simulink model "SafetyTemperatureSwitch"  (R2016b)
settings: Solver=FixedStepDiscrete  StartTime=0.0  StopTime=inf  RelTol=1e-3  EnableMultiTasking=on
settings Model: xpc_rtwmakecfg_data=_xpcethercatlib_  Creator=march  LastModifiedBy=march
settings SolverCC: EnableConcurrentExecution=on  AutoInsertRateTranBlk=on
settings DataIOCC: SaveFormat=StructureWithTime  SaveOutput=off  SaveTime=off
settings OptimizationCC: BlockReduction=off  OptimizeBlockIOStorage=off  BufferReuse=off  GlobalBufferReuse=off  ExpressionFolding=off  LocalBlockOutputs=off
settings HardwareCC: ProdBitPerPointer=32  ProdBitPerSizeT=32  ProdBitPerPtrDiffT=32  ProdLargestAtomicFloat=None  ProdWordSize=32  ProdLongLongMode=on  ProdHWDeviceType=Generic->32-bit x86 compatible
settings RTWCC: SystemTargetFile=slrt.tlc  TemplateMakefile=slrt_default_tmf  PostCodeGenCommand=SomanetTuning_make_rtw_hook  Description=Simulink Real-Time  RTWVerbose=off  CodeExecutionProfiling=on  RTWCompilerOptimization=on
settings SimulinkRealTimeCC: xPCModelTimeoutSecs=20

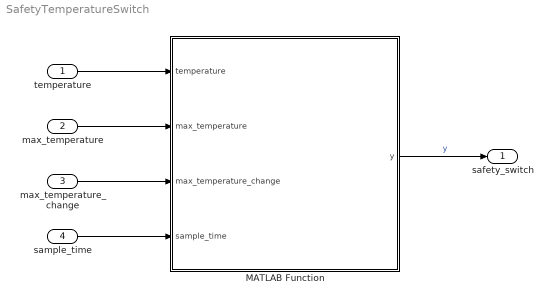
== system SafetyTemperatureSwitch ==
  "temperature " : Inport
  max_temperature : Inport  Port=2
  max_temperature_change : Inport  Port=3
  sample_time : Inport  Port=4
  MATLAB Function : MATLAB Function  TreatAsAtomicUnit=on
  safety_switch : Outport
  wires:
  sample_time/1 -> MATLAB Function/4(sample_time)
  max_temperature_change/1 -> MATLAB Function/3(max_temperature_change)
  max_temperature/1 -> MATLAB Function/2(max_temperature)
  "temperature "/1 -> MATLAB Function/1(temperature)
  MATLAB Function/1(y) -> safety_switch/1  "y"

== matlab function SafetyTemperatureSwitch/MATLAB Function ==
  data: temperature input; y output; max_temperature input; max_temperature_change input; sample_time input
function y = func_temperature_switch(temperature,max_temperature, max_temperature_change, sample_time)

    persistent last_temp
    persistent time_out
    
    if (isempty(last_temp))
        last_temp = 0;              % the temperature 0 to 0.5 seconds ago.
        time_out = 0;               % temperature is 'measured' every half second to check change over time
      
    end
    
            
    %sets output to true if temperature exceeds max temperature
    if temperature > max_temperature 
        y = true;
        
        time_out = 60/sample_time; %ensures a full stop for 60seconds once limits are exceeded

                
    %sets output to true if temperature changes too much per second
    elseif   last_temp > 30 && (temperature-last_temp)/0.5 > max_temperature_change  
        y = true;
        
        time_out = 60/sample_time;  %ensures a full stop for 60seconds once limits are exceeded
        
        
        
        %keeps quick stop activated for the intended 60 seconds during time out
    elseif time_out > 0.5 / sample_time 
       
        y = true;
        
    else
        % if noting is wrong keeps somanet on
        y = false;
        
    end
    
    %remembers the temperature every half second so that the temperature
    %change can be checked.
    if time_out == 0
        
        last_temp = double(temperature);
        time_out = 0.5 / sample_time;
    else
        time_out = time_out  - 1;
    end


end
